simulink model "NE_Red_Rooster_Delta_B_28may"  (R2019b)
settings: Solver=FixedStepAuto  StartTime=0.0  StopTime=inf  FixedStep=0.0005  RelTol=1e-3
PreLoadFcn:
  | waijung.modelPreload; % Required for working with Waijung Blockset. Do not remove.
undefined symbols (not defined in the file): ARM, DiscIntNeverNeededParam, HSEOSC, Link, LQFP100, MDK, ST, STM32F407VG
libraries: simulink x30, stm32f4_i2c_lib x22, stm32f4_io_lib x6, stm32f4_reset_lib x1, stm32f4_device_config_lib x1
(part 4 of 5)

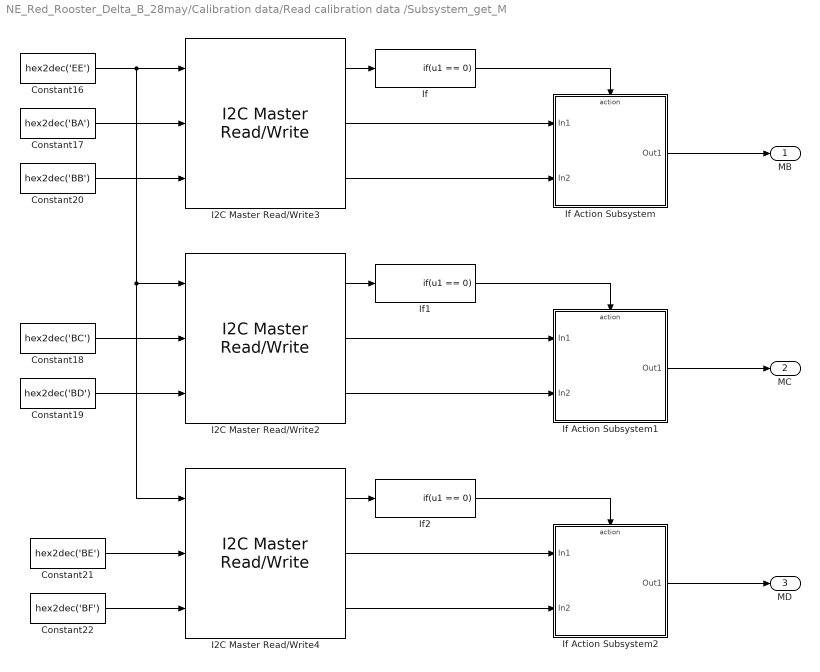
== system NE_Red_Rooster_Delta_B_28may/Calibration data/Read calibration data /Subsystem_get_M ==
  Constant16 : Constant  Value=hex2dec('EE')  OutDataTypeStr=uint8
  Constant17 : Constant  Value=hex2dec('BA')  OutDataTypeStr=uint8
  Constant18 : Constant  Value=hex2dec('BC')  OutDataTypeStr=uint8
  Constant19 : Constant  Value=hex2dec('BD')  OutDataTypeStr=uint8
  Constant20 : Constant  Value=hex2dec('BB')  OutDataTypeStr=uint8
  Constant21 : Constant  Value=hex2dec('BE')  OutDataTypeStr=uint8
  Constant22 : Constant  Value=hex2dec('BF')  OutDataTypeStr=uint8
  I2C Master Read/Write2 : stm32f4_i2c_lib/I2C Master Read//Write  configuration=Transaction  module=1  lastmodule=3  transfer=Blocking  dutycycle=TLow/THigh = 2  clkspeed=400  timeout=25  writecount=2  readcount=2  sdapin=C9  sclpin=A8  waitwritetime=0  forcestop=off  inputtypearray=[3 3 3 3]  outputtypearray=[3 3 3 3]  confstr="[\"C\",\"9\",\"A\",\"8\",\"1\",\"1\",\"6\",\"0\",\"I2C_DutyCycle_2\",\"0\",\"off\"]"  sampletime=-1  sampletimestr=Inf  blockid=CalibrationdataReadcalibrationdataSubsystem_get_MI2CMasterReadWrite2
  I2C Master Read/Write3 : stm32f4_i2c_lib/I2C Master Read//Write  configuration=Transaction  module=1  lastmodule=3  transfer=Blocking  dutycycle=TLow/THigh = 2  clkspeed=400  timeout=25  writecount=2  readcount=2  sdapin=C9  sclpin=A8  waitwritetime=0  forcestop=off  inputtypearray=[3 3 3 3]  outputtypearray=[3 3 3 3]  confstr="[\"C\",\"9\",\"A\",\"8\",\"1\",\"1\",\"6\",\"0\",\"I2C_DutyCycle_2\",\"0\",\"off\"]"  sampletime=-1  sampletimestr=Inf  blockid=CalibrationdataReadcalibrationdataSubsystem_get_MI2CMasterReadWrite3
  I2C Master Read/Write4 : stm32f4_i2c_lib/I2C Master Read//Write  configuration=Transaction  module=1  lastmodule=3  transfer=Blocking  dutycycle=TLow/THigh = 2  clkspeed=400  timeout=25  writecount=2  readcount=2  sdapin=C9  sclpin=A8  waitwritetime=0  forcestop=off  inputtypearray=[3 3 3 3]  outputtypearray=[3 3 3 3]  confstr="[\"C\",\"9\",\"A\",\"8\",\"1\",\"1\",\"6\",\"0\",\"I2C_DutyCycle_2\",\"0\",\"off\"]"  sampletime=-1  sampletimestr=Inf  blockid=CalibrationdataReadcalibrationdataSubsystem_get_MI2CMasterReadWrite4
  If : If  IfExpression=u1 == 0  ShowElse=off
  If Action Subsystem : Subsystem  TreatAsAtomicUnit=on
  If Action Subsystem1 : Subsystem  TreatAsAtomicUnit=on
  If Action Subsystem2 : Subsystem  TreatAsAtomicUnit=on
  If1 : If  IfExpression=u1 == 0  ShowElse=off
  If2 : If  IfExpression=u1 == 0  ShowElse=off
  MB : Outport
  MC : Outport  Port=2
  MD : Outport  Port=3
  wires:
  If Action Subsystem1/1(Out1) -> MC/1
  I2C Master Read/Write2/3 -> If Action Subsystem1/2(In2)
  I2C Master Read/Write3/1 -> If/1
  Constant16/1 -> I2C Master Read/Write4/1, I2C Master Read/Write2/1, I2C Master Read/Write3/1
  Constant22/1 -> I2C Master Read/Write4/3
  Constant21/1 -> I2C Master Read/Write4/2
  Constant20/1 -> I2C Master Read/Write3/3
  Constant18/1 -> I2C Master Read/Write2/2
  I2C Master Read/Write4/1 -> If2/1
  If1/1 -> If Action Subsystem1/Action
  If/1 -> If Action Subsystem/Action
  Constant19/1 -> I2C Master Read/Write2/3
  I2C Master Read/Write3/2 -> If Action Subsystem/1(In1)
  Constant17/1 -> I2C Master Read/Write3/2
  I2C Master Read/Write4/3 -> If Action Subsystem2/2(In2)
  I2C Master Read/Write3/3 -> If Action Subsystem/2(In2)
  If Action Subsystem/1(Out1) -> MB/1
  I2C Master Read/Write2/2 -> If Action Subsystem1/1(In1)
  I2C Master Read/Write4/2 -> If Action Subsystem2/1(In1)
  If Action Subsystem2/1(Out1) -> MD/1
  If2/1 -> If Action Subsystem2/Action
  I2C Master Read/Write2/1 -> If1/1

== system NE_Red_Rooster_Delta_B_28may/Init_L3GD4200 /Init L3G4200D/Subsystem ==
  Enable : EnablePort
  Logical Operator : Logic  Operator=NOT  AllPortsSameDT=off  OutDataTypeStr=boolean
  Memory : Memory  InheritSampleTime=on
  Out1 : Outport
  wires:
  Logical Operator/1 -> Out1/1, Memory/1
  Memory/1 -> Logical Operator/1

== system NE_Red_Rooster_Delta_B_28may/Init_L3GD4200 /Init L3G4200D/Subsystem1 ==
  Enable : EnablePort
  Logical Operator : Logic  Operator=NOT  AllPortsSameDT=off  OutDataTypeStr=boolean
  Memory : Memory  InheritSampleTime=on
  Out1 : Outport
  wires:
  Memory/1 -> Logical Operator/1
  Logical Operator/1 -> Memory/1, Out1/1

== system NE_Red_Rooster_Delta_B_28may/Orientation/Accelerometr/Manipulate Data ==
  LowAddress : Inport
  HighAddress : Inport  Port=2
  Add : Sum
  Data Type Conversion : DataTypeConversion  OutDataTypeStr=int16
  Data Type Conversion1 : DataTypeConversion  OutDataTypeStr=int16
  Shift Arithmetic1 : ArithShift  BitShiftNumber=8  BitShiftDirection=Left
  RawAccData : Outport
  wires:
  LowAddress/1 -> Data Type Conversion/1
  HighAddress/1 -> Data Type Conversion1/1
  Data Type Conversion/1 -> Add/1
  Data Type Conversion1/1 -> Shift Arithmetic1/1
  Shift Arithmetic1/1 -> Add/2
  Add/1 -> RawAccData/1

== system NE_Red_Rooster_Delta_B_28may/Orientation/Accelerometr/Manipulate Data1 ==
  LowAddress : Inport
  HighAddress : Inport  Port=2
  Add : Sum
  Data Type Conversion : DataTypeConversion  OutDataTypeStr=int16
  Data Type Conversion1 : DataTypeConversion  OutDataTypeStr=int16
  Shift Arithmetic1 : ArithShift  BitShiftNumber=8  BitShiftDirection=Left
  RawAccData : Outport
  wires:
  Add/1 -> RawAccData/1
  Shift Arithmetic1/1 -> Add/2
  Data Type Conversion1/1 -> Shift Arithmetic1/1
  Data Type Conversion/1 -> Add/1
  HighAddress/1 -> Data Type Conversion1/1
  LowAddress/1 -> Data Type Conversion/1

== system NE_Red_Rooster_Delta_B_28may/Orientation/Accelerometr/Manipulate Data2 ==
  LowAddress : Inport
  HighAddress : Inport  Port=2
  Add : Sum
  Data Type Conversion : DataTypeConversion  OutDataTypeStr=int16
  Data Type Conversion1 : DataTypeConversion  OutDataTypeStr=int16
  Shift Arithmetic1 : ArithShift  BitShiftNumber=8  BitShiftDirection=Left
  RawAccData : Outport
  wires:
  LowAddress/1 -> Data Type Conversion/1
  HighAddress/1 -> Data Type Conversion1/1
  Data Type Conversion/1 -> Add/1
  Data Type Conversion1/1 -> Shift Arithmetic1/1
  Shift Arithmetic1/1 -> Add/2
  Add/1 -> RawAccData/1

== system NE_Red_Rooster_Delta_B_28may/Orientation/Accelerometr/Subsystem ==
  Enable : EnablePort
  Logical Operator : Logic  Operator=NOT  AllPortsSameDT=off  OutDataTypeStr=boolean
  Memory : Memory  InheritSampleTime=on
  Out1 : Outport
  wires:
  Logical Operator/1 -> Out1/1, Memory/1
  Memory/1 -> Logical Operator/1

== system NE_Red_Rooster_Delta_B_28may/Orientation/Accelerometr/Subsystem1 ==
  Enable : EnablePort
  Logical Operator : Logic  Operator=NOT  AllPortsSameDT=off  OutDataTypeStr=boolean
  Memory : Memory  InheritSampleTime=on
  Out1 : Outport
  wires:
  Memory/1 -> Logical Operator/1
  Logical Operator/1 -> Memory/1, Out1/1

== system NE_Red_Rooster_Delta_B_28may/Orientation/Accelerometr/Subsystem2 ==
  Enable : EnablePort
  Logical Operator : Logic  Operator=NOT  AllPortsSameDT=off  OutDataTypeStr=boolean
  Memory : Memory  InheritSampleTime=on
  Out1 : Outport
  wires:
  Logical Operator/1 -> Out1/1, Memory/1
  Memory/1 -> Logical Operator/1

== system NE_Red_Rooster_Delta_B_28may/Orientation/Gyro/Data_transformation ==
  In1 : Inport
  In2 : Inport  Port=2
  In3 : Inport  Port=3
  Gain : Gain  Gain=5
  Gain1 : Gain  Gain=5
  Gain2 : Gain  Gain=5
  Subsystem : Subsystem
  Subsystem1 : Subsystem
  Subsystem2 : Subsystem
  Subsystem3 : Subsystem
  Out1 : Outport
  Out2 : Outport  Port=2
  Out3 : Outport  Port=3
  wires:
  Subsystem2/1(Out1) -> Out1/1
  Subsystem2/2(Out2) -> Out2/1
  Subsystem2/3(Out3) -> Out3/1
  In1/1 -> Subsystem/1(In1)
  In2/1 -> Subsystem1/1(In1)
  In3/1 -> Subsystem3/1(In1)
  Subsystem/1(Grad/sek) -> Gain/1
  Subsystem1/1(Grad/sek) -> Gain1/1
  Subsystem3/1(Grad/sek) -> Gain2/1
  Gain/1 -> Subsystem2/1(In1)
  Gain1/1 -> Subsystem2/2(In2)
  Gain2/1 -> Subsystem2/3(In3)

== system NE_Red_Rooster_Delta_B_28may/Orientation/Gyro/L3G4200D ==
  Read L3G4200D : Subsystem  TreatAsAtomicUnit=on
  SlvAddr1 : Constant  Value=hex2dec('D2')  OutDataTypeStr=uint8  SampleTime=-1
  Status : Outport
  X : Outport  Port=2
  Y : Outport  Port=3
  Z : Outport  Port=4
  wires:
  Read L3G4200D/4(OUT_Z) -> Z/1
  Read L3G4200D/3(OUT_Y) -> Y/1
  Read L3G4200D/2(OUT_X) -> X/1
  Read L3G4200D/1(Status) -> Status/1
  SlvAddr1/1 -> Read L3G4200D/1(SlvAddr)

== system NE_Red_Rooster_Delta_B_28may/Orientation/Gyro/Success ==
  In1 : Inport
  In2 : Inport  Port=2
  In3 : Inport  Port=3
  Enable : EnablePort  PropagateVarSize=During execution
  Data Type Conversion : DataTypeConversion  OutDataTypeStr=int16
  Demux : Demux  Outputs=3
  Gain : Gain  Gain=250/2^15  ParamDataTypeStr=single  OutDataTypeStr=single
  Mux : Mux  Inputs=3
  Gyr_X : Outport
  Gyr_Y : Outport  Port=2
  Gyr_Z : Outport  Port=3
  wires:
  Data Type Conversion/1 -> Gain/1
  In3/1 -> Mux/3
  In2/1 -> Mux/2
  In1/1 -> Mux/1
  Demux/3 -> Gyr_Z/1
  Demux/2 -> Gyr_Y/1
  Demux/1 -> Gyr_X/1
  Gain/1 -> Demux/1
  Mux/1 -> Data Type Conversion/1

== system NE_Red_Rooster_Delta_B_28may/Baro_Altimeter/Calculate true pressure and temp /Calculate true pressure1/Altitude ==
  In1 : Inport
  "Null_Pressure " : Inport  Port=2
  Constant : Constant  Value=44330  OutDataTypeStr=int32
  Constant1 : Constant  OutDataTypeStr=int32
  Constant2 : Constant  Value=0.19  OutDataTypeStr=double
  Constant3 : Constant  Value=102159
  Divide : Product  Inputs=*/  OutDataTypeStr=double
  Math Function : Math  Operator=pow  SaturateOnIntegerOverflow=on
  Product : Product  OutDataTypeStr=single
  Subtract : Sum  Inputs=+-  OutDataTypeStr=double
  Terminator : Terminator
  Out1 : Outport
  wires:
  Product/1 -> Out1/1
  Constant1/1 -> Subtract/1
  Constant/1 -> Product/2
  Constant2/1 -> Math Function/2
  Subtract/1 -> Product/1
  In1/1 -> Divide/1
  Divide/1 -> Math Function/1
  Math Function/1 -> Subtract/2
  "Null_Pressure "/1 -> Divide/2
  Constant3/1 -> Terminator/1

== system NE_Red_Rooster_Delta_B_28may/Baro_Altimeter/Calculate true pressure and temp /Calculate true pressure1/If Action Subsystem ==
  B7 : Inport
  B4 : Inport  Port=2
  Action Port : ActionPort  ActionPortLabel=if { }
  Constant : Constant  Value=2  OutDataTypeStr=uint32
  Divide : Product  Inputs=*/  OutDataTypeStr=uint32
  Product : Product  OutDataTypeStr=uint32
  p : Outport  OutDataTypeStr=uint32
  wires:
  B7/1 -> Product/1
  Constant/1 -> Product/2
  Product/1 -> Divide/1
  B4/1 -> Divide/2
  Divide/1 -> p/1

== system NE_Red_Rooster_Delta_B_28may/Baro_Altimeter/Calculate true pressure and temp /Calculate true pressure1/If Action Subsystem1 ==
  B7 : Inport
  B4 : Inport  Port=2
  Action Port : ActionPort  ActionPortLabel=else { }
  Constant : Constant  Value=2  OutDataTypeStr=uint32
  Divide : Product  Inputs=*/
  Product : Product  OutDataTypeStr=uint32
  p : Outport  OutDataTypeStr=uint32
  wires:
  Constant/1 -> Product/2
  B4/1 -> Divide/2
  B7/1 -> Divide/1
  Divide/1 -> Product/1
  Product/1 -> p/1

== system NE_Red_Rooster_Delta_B_28may/Baro_Altimeter/Calculate true pressure and temp /Calculate true pressure1/New X1 value ==
  note: Версия 1: Формула для вычисления X1 имела следующий вид:
      | X1=AC3*B6/2^13
      | Я сначало делил потом умножал...
      |
      | Версия 2: X1=(AC3*B6)/2^13. Теперь я умножаю,а потом делю
  B6 : Inport
  AC3 : Inport  Port=2
  Constant : Constant  Value=8192  OutDataTypeStr=int32
  Divide : Product  Inputs=*/
  Product : Product  OutDataTypeStr=int32
  X1_1 : Outport  OutDataTypeStr=int32
  wires:
  AC3/1 -> Product/1
  Constant/1 -> Divide/2
  Product/1 -> Divide/1
  B6/1 -> Product/2
  Divide/1 -> X1_1/1

== system NE_Red_Rooster_Delta_B_28may/Baro_Altimeter/Calculate true pressure and temp /Calculate true pressure1/New_X2 ==
  B6 : Inport
  B1 : Inport  Port=2
  Constant1 : Constant  Value=4096  OutDataTypeStr=int32
  Constant2 : Constant  Value=65536  OutDataTypeStr=int32
  Divide : Product  Inputs=*/  OutDataTypeStr=int32
  Divide1 : Product  Inputs=*/  OutDataTypeStr=int32
  Product : Product  OutDataTypeStr=int32
  Product1 : Product  OutDataTypeStr=int32
  X2_1 : Outport  OutDataTypeStr=int32
  wires:
  B1/1 -> Product1/2
  Constant1/1 -> Divide/2
  B6/1 -> Product/2, Product/1
  Product1/1 -> Divide1/1
  Constant2/1 -> Divide1/2
  Divide1/1 -> X2_1/1
  Product/1 -> Divide/1
  Divide/1 -> Product1/1

== system NE_Red_Rooster_Delta_B_28may/Baro_Altimeter/Calculate true pressure and temp /Calculate true pressure1/Sub ==
  B6 : Inport
  B2 : Inport  Port=2
  2e11 : Subsystem
  2e12 : Subsystem
  Divide : Product  Inputs=*/
  Divide1 : Product  Inputs=*/
  Math Function : Math  Operator=square  SaturateOnIntegerOverflow=on
  Product1 : Product
  X1 : Outport
  wires:
  Divide1/1 -> X1/1
  2e11/1(Out1) -> Divide1/2
  Product1/1 -> Divide1/1
  B6/1 -> Math Function/1
  2e12/1(Out1) -> Divide/2
  B2/1 -> Product1/2
  Math Function/1 -> Divide/1
  Divide/1 -> Product1/1

== system NE_Red_Rooster_Delta_B_28may/Baro_Altimeter/Calculate true pressure and temp /Calculate true pressure1/Subsystem ==
  B5 : Inport
  Constant : Constant  Value=4000  OutDataTypeStr=int32
  Subtract : Sum  Inputs=+-  OutDataTypeStr=int32
  B6 : Outport  OutDataTypeStr=int32
  wires:
  B5/1 -> Subtract/1
  Subtract/1 -> B6/1
  Constant/1 -> Subtract/2

== system NE_Red_Rooster_Delta_B_28may/Baro_Altimeter/Calculate true pressure and temp /Calculate true pressure1/Subsystem1 ==
  B6 : Inport
  AC2 : Inport  Port=2
  2e11 : Subsystem
  Divide : Product  Inputs=*/
  Product : Product
  X2 : Outport
  wires:
  B6/1 -> Divide/1
  Product/1 -> X2/1
  Divide/1 -> Product/2
  2e11/1(Out1) -> Divide/2
  AC2/1 -> Product/1

== system NE_Red_Rooster_Delta_B_28may/Baro_Altimeter/Calculate true pressure and temp /Calculate true pressure1/Subsystem2 ==
  note: В тестовом примере сдвиг равен нулю, а у нас 3, с этого момента начинает алгоритм плыть..
  X3 : Inport
  AC1 : Inport  Port=2
  Add1 : Sum  OutDataTypeStr=int32
  Add2 : Sum  AccumDataTypeStr=int32
  Constant : Constant  Value=4  OutDataTypeStr=int32
  Constant1 : Constant  Value=2  OutDataTypeStr=int32
  Constant2 : Constant  Value=4  OutDataTypeStr=int32
  Divide : Product  Inputs=*/  OutDataTypeStr=int32
  Product : Product  OutDataTypeStr=int32
  Shift Arithmetic7 : ArithShift  BitShiftNumber=3  BitShiftDirection=Left  DiagnosticForOORShift=Warning
  B3 : Outport  OutDataTypeStr=int32
  wires:
  X3/1 -> Add1/1
  Product/1 -> Add1/2
  Constant/1 -> Product/2
  Divide/1 -> B3/1
  Constant2/1 -> Divide/2
  Shift Arithmetic7/1 -> Add2/1
  Add1/1 -> Shift Arithmetic7/1
  Add2/1 -> Divide/1
  Constant1/1 -> Add2/2
  AC1/1 -> Product/1

== system NE_Red_Rooster_Delta_B_28may/Baro_Altimeter/Calculate true pressure and temp /Calculate true pressure1/Subsystem3 ==
  X1_1 : Inport
  X2_1 : Inport  Port=2
  Add1 : Sum
  Add2 : Sum  AccumDataTypeStr=int32
  Constant : Constant  Value=2  OutDataTypeStr=int32
  Constant1 : Constant  Value=4  OutDataTypeStr=int32
  Divide : Product  Inputs=*/  OutDataTypeStr=int32
  X3_1 : Outport  OutDataTypeStr=int32
  wires:
  Divide/1 -> X3_1/1
  X1_1/1 -> Add1/1
  Constant1/1 -> Divide/2
  Add2/1 -> Divide/1
  Constant/1 -> Add2/2
  X2_1/1 -> Add1/2
  Add1/1 -> Add2/1

== system NE_Red_Rooster_Delta_B_28may/Baro_Altimeter/Calculate true pressure and temp /Calculate true pressure1/Subsystem4 ==
  X3_1 : Inport
  AC4 : Inport  Port=2
  Add1 : Sum  OutDataTypeStr=uint32
  Constant : Constant  Value=32768  OutDataTypeStr=uint32
  Constant1 : Constant  Value=32768  OutDataTypeStr=uint32
  Divide : Product  Inputs=*/  OutDataTypeStr=uint32
  Product : Product  OutDataTypeStr=uint32
  B4 : Outport  OutDataTypeStr=uint32
  wires:
  AC4/1 -> Product/2
  X3_1/1 -> Add1/1
  Constant/1 -> Add1/2
  Constant1/1 -> Divide/2
  Add1/1 -> Product/1
  Product/1 -> Divide/1
  Divide/1 -> B4/1

== system NE_Red_Rooster_Delta_B_28may/Baro_Altimeter/Calculate true pressure and temp /Calculate true pressure1/Subsystem5 ==
  B3 : Inport
  UP : Inport  Port=2
  Constant : Constant  Value=50000  OutDataTypeStr=uint32
  Product : Product  OutDataTypeStr=uint32
  Shift Arithmetic7 : ArithShift  BitShiftNumber=2  BitShiftDirection=Right
  Subtract : Sum  Inputs=+-
  B7 : Outport  OutDataTypeStr=uint32
  wires:
  Constant/1 -> Shift Arithmetic7/1
  UP/1 -> Subtract/1
  Shift Arithmetic7/1 -> Product/2
  B3/1 -> Subtract/2
  Subtract/1 -> Product/1
  Product/1 -> B7/1

== system NE_Red_Rooster_Delta_B_28may/Baro_Altimeter/Calculate true pressure and temp /Calculate true pressure1/Subsystem6 ==
  p : Inport
  Constant : Constant  Value=256  OutDataTypeStr=uint32
  Constant1 : Constant  Value=256  OutDataTypeStr=uint32
  Divide : Product  Inputs=*/  OutDataTypeStr=uint32
  Divide1 : Product  Inputs=*/  OutDataTypeStr=uint32
  Product : Product  OutDataTypeStr=uint32
  X1 : Outport  OutDataTypeStr=uint32
  wires:
  Constant1/1 -> Divide1/2
  p/1 -> Divide1/1, Divide/1
  Constant/1 -> Divide/2
  Divide/1 -> Product/1
  Product/1 -> X1/1
  Divide1/1 -> Product/2

== system NE_Red_Rooster_Delta_B_28may/Baro_Altimeter/Calculate true pressure and temp /Calculate true pressure1/Subsystem7 ==
  X1 : Inport
  Constant : Constant  Value=3038  OutDataTypeStr=uint32
  Constant1 : Constant  Value=65536  OutDataTypeStr=uint32
  Divide : Product  Inputs=*/  OutDataTypeStr=uint32
  Product : Product
  X1_1 : Outport  OutDataTypeStr=uint32
  wires:
  X1/1 -> Product/1
  Product/1 -> Divide/1
  Constant1/1 -> Divide/2
  Divide/1 -> X1_1/1
  Constant/1 -> Product/2

== system NE_Red_Rooster_Delta_B_28may/Baro_Altimeter/Calculate true pressure and temp /Calculate true pressure1/Subsystem8 ==
  p : Inport
  Constant : Constant  Value=-7357  OutDataTypeStr=int32
  Constant1 : Constant  Value=65536  OutDataTypeStr=int32
  Divide : Product  Inputs=*/  OutDataTypeStr=int32
  Product : Product  OutDataTypeStr=int32
  X2 : Outport  OutDataTypeStr=int32
  wires:
  Product/1 -> Divide/1
  Constant1/1 -> Divide/2
  p/1 -> Product/1
  Divide/1 -> X2/1
  Constant/1 -> Product/2

== system NE_Red_Rooster_Delta_B_28may/Baro_Altimeter/Calculate true pressure and temp /Calculate true pressure1/Subsystem9 ==
  p : Inport
  X1_1 : Inport  Port=2
  X2 : Inport  Port=3
  Add1 : Sum  Inputs=+++  OutDataTypeStr=int32
  Add2 : Sum  OutDataTypeStr=int32
  Constant : Constant  Value=3791  OutDataTypeStr=uint32
  Constant1 : Constant  Value=16  OutDataTypeStr=uint32
  Divide : Product  Inputs=*/  OutDataTypeStr=int32
  p_1 : Outport  OutDataTypeStr=int32
  wires:
  X1_1/1 -> Add1/1
  X2/1 -> Add1/2
  Add1/1 -> Divide/1
  Constant/1 -> Add1/3
  Constant1/1 -> Divide/2
  Divide/1 -> Add2/2
  p/1 -> Add2/1
  Add2/1 -> p_1/1

== system NE_Red_Rooster_Delta_B_28may/Baro_Altimeter/Calculate true pressure and temp /Calculate true temperature1/Subsystem ==
  UT : Inport
  AC6 : Inport  Port=2
  AC5 : Inport  Port=3
  Add : Sum  Inputs=+-  OutDataTypeStr=int32
  Constant : Constant  Value=32768  OutDataTypeStr=int32
  Divide : Product  Inputs=*/  OutDataTypeStr=int32
  Product : Product
  X1 : Outport
  wires:
  AC6/1 -> Add/2
  UT/1 -> Add/1
  Add/1 -> Product/1
  Constant/1 -> Divide/2
  AC5/1 -> Product/2
  Product/1 -> Divide/1
  Divide/1 -> X1/1

== system NE_Red_Rooster_Delta_B_28may/Baro_Altimeter/Calculate true pressure and temp /Calculate true temperature1/Subsystem1 ==
  X1 : Inport
  MC : Inport  Port=2
  MD : Inport  Port=3
  Add : Sum
  Constant2 : Constant  Value=2048  OutDataTypeStr=int32
  Divide : Product  Inputs=*/  OutDataTypeStr=int32
  Product : Product  OutDataTypeStr=int32
  X2 : Outport
  wires:
  Divide/1 -> X2/1
  X1/1 -> Add/1
  Add/1 -> Divide/2
  MD/1 -> Add/2
  Product/1 -> Divide/1
  MC/1 -> Product/1
  Constant2/1 -> Product/2

== system NE_Red_Rooster_Delta_B_28may/Baro_Altimeter/Calculate true pressure and temp /Calculate true temperature1/Subsystem2 ==
  B5 : Inport
  Add1 : Sum  OutDataTypeStr=int32
  Constant : Constant  Value=8  OutDataTypeStr=uint32
  Constant1 : Constant  Value=16
  Divide : Product  Inputs=*/  OutDataTypeStr=int32
  T : Outport  OutDataTypeStr=int32
  wires:
  B5/1 -> Add1/1
  Add1/1 -> Divide/1
  Constant/1 -> Add1/2
  Constant1/1 -> Divide/2
  Divide/1 -> T/1

== system NE_Red_Rooster_Delta_B_28may/Baro_Altimeter/Read Pressure and Temp/If Action Subsystem/If Action Subsystem ==
  In1 : Inport
  Action Port : ActionPort  ActionPortLabel=if { }
  Data Type Conversion15 : DataTypeConversion  OutDataTypeStr=uint32
  Out1 : Outport
  wires:
  Data Type Conversion15/1 -> Out1/1
  In1/1 -> Data Type Conversion15/1

== system NE_Red_Rooster_Delta_B_28may/Baro_Altimeter/Read Pressure and Temp/If Action Subsystem/If Action Subsystem1 ==
  In1 : Inport
  Action Port : ActionPort  ActionPortLabel=if { }
  Constant : Constant  Value=16777216  OutDataTypeStr=uint32  SampleTime=-1
  Subtract : Sum  Inputs=+-  OutDataTypeStr=int32
  Out1 : Outport
  wires:
  In1/1 -> Subtract/1
  Subtract/1 -> Out1/1
  Constant/1 -> Subtract/2

== system NE_Red_Rooster_Delta_B_28may/Baro_Altimeter/Read Pressure and Temp/If Action Subsystem/If Action Subsystem2 ==
  In1 : Inport
  Action Port : ActionPort  ActionPortLabel=else { }
  Out1 : Outport
  wires:
  In1/1 -> Out1/1

== system NE_Red_Rooster_Delta_B_28may/Baro_Altimeter/Read Pressure and Temp/If Action Subsystem/If Action Subsystem3 ==
  In1 : Inport
  Action Port : ActionPort  ActionPortLabel=if { }
  Data Type Conversion15 : DataTypeConversion  OutDataTypeStr=uint32
  Out1 : Outport
  wires:
  Data Type Conversion15/1 -> Out1/1
  In1/1 -> Data Type Conversion15/1

== system NE_Red_Rooster_Delta_B_28may/Baro_Altimeter/Read Pressure and Temp/If Action Subsystem2/If Action Subsystem ==
  In1 : Inport
  Action Port : ActionPort  ActionPortLabel=if { }
  Data Type Conversion4 : DataTypeConversion  OutDataTypeStr=uint32
  Out1 : Outport
  wires:
  In1/1 -> Data Type Conversion4/1
  Data Type Conversion4/1 -> Out1/1

== system NE_Red_Rooster_Delta_B_28may/Baro_Altimeter/Read Pressure and Temp/If Action Subsystem2/If Action Subsystem1 ==
  In2 : Inport
  Action Port : ActionPort  ActionPortLabel=if { }
  Data Type Conversion1 : DataTypeConversion  OutDataTypeStr=uint32
  Out1 : Outport
  wires:
  In2/1 -> Data Type Conversion1/1
  Data Type Conversion1/1 -> Out1/1

== system NE_Red_Rooster_Delta_B_28may/Baro_Altimeter/Read Pressure and Temp/If Action Subsystem2/If Action Subsystem2 ==
  In2 : Inport
  Action Port : ActionPort  ActionPortLabel=if { }
  Data Type Conversion1 : DataTypeConversion  OutDataTypeStr=uint32
  Out1 : Outport
  wires:
  In2/1 -> Data Type Conversion1/1
  Data Type Conversion1/1 -> Out1/1

== system NE_Red_Rooster_Delta_B_28may/Calibration data/Read calibration data /Subsystem_get_AC/If Action Subsystem ==
  In1 : Inport
  In2 : Inport  Port=2
  Action Port : ActionPort  ActionPortLabel=if { }
  Add9 : Sum  AccumDataTypeStr=uint32  OutDataTypeStr=int32
  Compare To Constant : simulink/Logic and Bit Operations/Compare To Constant  relop=>=  const=128  OutDataTypeStr=boolean
  Data Type Conversion15 : DataTypeConversion  OutDataTypeStr=uint32
  Data Type Conversion16 : DataTypeConversion  OutDataTypeStr=uint32
  If : If  IfExpression=u1 >= 128
  If Action Subsystem : Subsystem  TreatAsAtomicUnit=on
  If Action Subsystem1 : Subsystem  TreatAsAtomicUnit=on
  Shift Arithmetic9 : ArithShift  BitShiftNumber=8  BitShiftDirection=Left
  Switch : Switch  Criteria=u2 > Threshold
  Out1 : Outport
  wires:
  Compare To Constant/1 -> Switch/2
  Switch/1 -> Out1/1
  If Action Subsystem1/1(Out1) -> Switch/3
  If Action Subsystem/1(Out1) -> Switch/1
  If/2 -> If Action Subsystem1/Action
  Add9/1 -> If Action Subsystem/1(In1), If Action Subsystem1/1(In1)
  If/1 -> If Action Subsystem/Action
  In2/1 -> Data Type Conversion16/1
  In1/1 -> Data Type Conversion15/1
  Data Type Conversion15/1 -> Shift Arithmetic9/1, If/1, Compare To Constant/1
  Data Type Conversion16/1 -> Add9/2
  Shift Arithmetic9/1 -> Add9/1

== system NE_Red_Rooster_Delta_B_28may/Calibration data/Read calibration data /Subsystem_get_AC/If Action Subsystem1 ==
  In1 : Inport
  In2 : Inport  Port=2
  Action Port : ActionPort  ActionPortLabel=if { }
  Add9 : Sum  AccumDataTypeStr=uint32  OutDataTypeStr=int32
  Compare To Constant : simulink/Logic and Bit Operations/Compare To Constant  relop=>=  const=128  OutDataTypeStr=boolean
  Data Type Conversion15 : DataTypeConversion  OutDataTypeStr=uint32
  Data Type Conversion16 : DataTypeConversion  OutDataTypeStr=uint32
  If : If  IfExpression=u1 >= 128
  If Action Subsystem : Subsystem  TreatAsAtomicUnit=on
  If Action Subsystem1 : Subsystem  TreatAsAtomicUnit=on
  Shift Arithmetic9 : ArithShift  BitShiftNumber=8  BitShiftDirection=Left
  Switch : Switch  Criteria=u2 > Threshold
  Out1 : Outport
  wires:
  Compare To Constant/1 -> Switch/2
  Switch/1 -> Out1/1
  If Action Subsystem1/1(Out1) -> Switch/3
  If Action Subsystem/1(Out1) -> Switch/1
  If/2 -> If Action Subsystem1/Action
  Add9/1 -> If Action Subsystem/1(In1), If Action Subsystem1/1(In1)
  If/1 -> If Action Subsystem/Action
  In2/1 -> Data Type Conversion16/1
  In1/1 -> Data Type Conversion15/1
  Data Type Conversion15/1 -> Shift Arithmetic9/1, If/1, Compare To Constant/1
  Data Type Conversion16/1 -> Add9/2
  Shift Arithmetic9/1 -> Add9/1

== system NE_Red_Rooster_Delta_B_28may/Calibration data/Read calibration data /Subsystem_get_AC/If Action Subsystem2 ==
  In1 : Inport
  In2 : Inport  Port=2
  Action Port : ActionPort  ActionPortLabel=if { }
  Add9 : Sum  AccumDataTypeStr=uint32  OutDataTypeStr=int32
  Compare To Constant : simulink/Logic and Bit Operations/Compare To Constant  relop=>=  const=128  OutDataTypeStr=boolean
  Data Type Conversion15 : DataTypeConversion  OutDataTypeStr=uint32
  Data Type Conversion16 : DataTypeConversion  OutDataTypeStr=uint32
  If : If  IfExpression=u1 >= 128
  If Action Subsystem : Subsystem  TreatAsAtomicUnit=on
  If Action Subsystem1 : Subsystem  TreatAsAtomicUnit=on
  Shift Arithmetic9 : ArithShift  BitShiftNumber=8  BitShiftDirection=Left
  Switch : Switch  Criteria=u2 > Threshold
  Out1 : Outport
  wires:
  Compare To Constant/1 -> Switch/2
  Switch/1 -> Out1/1
  If Action Subsystem1/1(Out1) -> Switch/3
  If Action Subsystem/1(Out1) -> Switch/1
  If/2 -> If Action Subsystem1/Action
  Add9/1 -> If Action Subsystem/1(In1), If Action Subsystem1/1(In1)
  If/1 -> If Action Subsystem/Action
  In2/1 -> Data Type Conversion16/1
  In1/1 -> Data Type Conversion15/1
  Data Type Conversion15/1 -> Shift Arithmetic9/1, If/1, Compare To Constant/1
  Data Type Conversion16/1 -> Add9/2
  Shift Arithmetic9/1 -> Add9/1

== system NE_Red_Rooster_Delta_B_28may/Calibration data/Read calibration data /Subsystem_get_AC/If Action Subsystem3 ==
  In1 : Inport
  In2 : Inport  Port=2
  Action Port : ActionPort  ActionPortLabel=if { }
  Add9 : Sum  AccumDataTypeStr=uint32  OutDataTypeStr=uint32
  Data Type Conversion15 : DataTypeConversion  OutDataTypeStr=uint32
  Data Type Conversion16 : DataTypeConversion  OutDataTypeStr=uint32
  Shift Arithmetic9 : ArithShift  BitShiftNumber=8  BitShiftDirection=Left
  Out1 : Outport
  wires:
  In2/1 -> Data Type Conversion16/1
  In1/1 -> Data Type Conversion15/1
  Data Type Conversion15/1 -> Shift Arithmetic9/1
  Data Type Conversion16/1 -> Add9/2
  Shift Arithmetic9/1 -> Add9/1
  Add9/1 -> Out1/1

== system NE_Red_Rooster_Delta_B_28may/Calibration data/Read calibration data /Subsystem_get_AC/If Action Subsystem4 ==
  In1 : Inport
  In2 : Inport  Port=2
  Action Port : ActionPort  ActionPortLabel=if { }
  Add9 : Sum  AccumDataTypeStr=uint32  OutDataTypeStr=uint32
  Data Type Conversion15 : DataTypeConversion  OutDataTypeStr=uint32
  Data Type Conversion16 : DataTypeConversion  OutDataTypeStr=uint32
  Shift Arithmetic9 : ArithShift  BitShiftNumber=8  BitShiftDirection=Left
  Out1 : Outport
  wires:
  In2/1 -> Data Type Conversion16/1
  In1/1 -> Data Type Conversion15/1
  Data Type Conversion15/1 -> Shift Arithmetic9/1
  Data Type Conversion16/1 -> Add9/2
  Shift Arithmetic9/1 -> Add9/1
  Add9/1 -> Out1/1

== system NE_Red_Rooster_Delta_B_28may/Calibration data/Read calibration data /Subsystem_get_AC/If Action Subsystem5 ==
  In1 : Inport
  In2 : Inport  Port=2
  Action Port : ActionPort  ActionPortLabel=if { }
  Add9 : Sum  AccumDataTypeStr=uint32  OutDataTypeStr=uint32
  Data Type Conversion15 : DataTypeConversion  OutDataTypeStr=uint32
  Data Type Conversion16 : DataTypeConversion  OutDataTypeStr=uint32
  Shift Arithmetic9 : ArithShift  BitShiftNumber=8  BitShiftDirection=Left
  Out1 : Outport
  wires:
  In2/1 -> Data Type Conversion16/1
  In1/1 -> Data Type Conversion15/1
  Data Type Conversion15/1 -> Shift Arithmetic9/1
  Data Type Conversion16/1 -> Add9/2
  Shift Arithmetic9/1 -> Add9/1
  Add9/1 -> Out1/1

== system NE_Red_Rooster_Delta_B_28may/Calibration data/Read calibration data /Subsystem_get_B/If Action Subsystem ==
  In1 : Inport
  In2 : Inport  Port=2
  Action Port : ActionPort  ActionPortLabel=if { }
  Add9 : Sum  AccumDataTypeStr=uint32  OutDataTypeStr=int32
  Compare To Constant : simulink/Logic and Bit Operations/Compare To Constant  relop=>=  const=128  OutDataTypeStr=boolean
  Data Type Conversion15 : DataTypeConversion  OutDataTypeStr=uint32
  Data Type Conversion16 : DataTypeConversion  OutDataTypeStr=uint32
  If : If  IfExpression=u1 >= 128
  If Action Subsystem : Subsystem  TreatAsAtomicUnit=on
  If Action Subsystem1 : Subsystem  TreatAsAtomicUnit=on
  Shift Arithmetic9 : ArithShift  BitShiftNumber=8  BitShiftDirection=Left
  Switch : Switch  Criteria=u2 > Threshold
  Out1 : Outport
  wires:
  Compare To Constant/1 -> Switch/2
  Switch/1 -> Out1/1
  If Action Subsystem1/1(Out1) -> Switch/3
  If Action Subsystem/1(Out1) -> Switch/1
  If/2 -> If Action Subsystem1/Action
  Add9/1 -> If Action Subsystem/1(In1), If Action Subsystem1/1(In1)
  If/1 -> If Action Subsystem/Action
  In2/1 -> Data Type Conversion16/1
  In1/1 -> Data Type Conversion15/1
  Data Type Conversion15/1 -> Shift Arithmetic9/1, If/1, Compare To Constant/1
  Data Type Conversion16/1 -> Add9/2
  Shift Arithmetic9/1 -> Add9/1

== system NE_Red_Rooster_Delta_B_28may/Calibration data/Read calibration data /Subsystem_get_B/If Action Subsystem1 ==
  In1 : Inport
  In2 : Inport  Port=2
  Action Port : ActionPort  ActionPortLabel=if { }
  Add9 : Sum  AccumDataTypeStr=uint32  OutDataTypeStr=int32
  Compare To Constant : simulink/Logic and Bit Operations/Compare To Constant  relop=>=  const=128  OutDataTypeStr=boolean
  Data Type Conversion15 : DataTypeConversion  OutDataTypeStr=uint32
  Data Type Conversion16 : DataTypeConversion  OutDataTypeStr=uint32
  If : If  IfExpression=u1 >= 128
  If Action Subsystem : Subsystem  TreatAsAtomicUnit=on
  If Action Subsystem1 : Subsystem  TreatAsAtomicUnit=on
  Shift Arithmetic9 : ArithShift  BitShiftNumber=8  BitShiftDirection=Left
  Switch : Switch  Criteria=u2 > Threshold
  Out1 : Outport
  wires:
  Compare To Constant/1 -> Switch/2
  Switch/1 -> Out1/1
  If Action Subsystem1/1(Out1) -> Switch/3
  If Action Subsystem/1(Out1) -> Switch/1
  If/2 -> If Action Subsystem1/Action
  Add9/1 -> If Action Subsystem/1(In1), If Action Subsystem1/1(In1)
  If/1 -> If Action Subsystem/Action
  In2/1 -> Data Type Conversion16/1
  In1/1 -> Data Type Conversion15/1
  Data Type Conversion15/1 -> Shift Arithmetic9/1, If/1, Compare To Constant/1
  Data Type Conversion16/1 -> Add9/2
  Shift Arithmetic9/1 -> Add9/1

== system NE_Red_Rooster_Delta_B_28may/Calibration data/Read calibration data /Subsystem_get_M/If Action Subsystem ==
  In1 : Inport
  In2 : Inport  Port=2
  Action Port : ActionPort  ActionPortLabel=if { }
  Add9 : Sum  AccumDataTypeStr=uint32  OutDataTypeStr=int32
  Compare To Constant : simulink/Logic and Bit Operations/Compare To Constant  relop=>=  const=128  OutDataTypeStr=boolean
  Data Type Conversion15 : DataTypeConversion  OutDataTypeStr=uint32
  Data Type Conversion16 : DataTypeConversion  OutDataTypeStr=uint32
  If : If  IfExpression=u1 >= 128
  If Action Subsystem : Subsystem  TreatAsAtomicUnit=on
  If Action Subsystem1 : Subsystem  TreatAsAtomicUnit=on
  Shift Arithmetic9 : ArithShift  BitShiftNumber=8  BitShiftDirection=Left
  Switch : Switch  Criteria=u2 > Threshold
  Out1 : Outport
  wires:
  Shift Arithmetic9/1 -> Add9/1
  Data Type Conversion16/1 -> Add9/2
  Data Type Conversion15/1 -> Compare To Constant/1, If/1, Shift Arithmetic9/1
  In1/1 -> Data Type Conversion15/1
  In2/1 -> Data Type Conversion16/1
  If/1 -> If Action Subsystem/Action
  Add9/1 -> If Action Subsystem1/1(In1), If Action Subsystem/1(In1)
  If/2 -> If Action Subsystem1/Action
  If Action Subsystem/1(Out1) -> Switch/1
  If Action Subsystem1/1(Out1) -> Switch/3
  Switch/1 -> Out1/1
  Compare To Constant/1 -> Switch/2

== system NE_Red_Rooster_Delta_B_28may/Calibration data/Read calibration data /Subsystem_get_M/If Action Subsystem1 ==
  In1 : Inport
  In2 : Inport  Port=2
  Action Port : ActionPort  ActionPortLabel=if { }
  Add9 : Sum  AccumDataTypeStr=uint32  OutDataTypeStr=int32
  Compare To Constant : simulink/Logic and Bit Operations/Compare To Constant  relop=>=  const=128  OutDataTypeStr=boolean
  Data Type Conversion15 : DataTypeConversion  OutDataTypeStr=uint32
  Data Type Conversion16 : DataTypeConversion  OutDataTypeStr=uint32
  If : If  IfExpression=u1 >= 128
  If Action Subsystem : Subsystem  TreatAsAtomicUnit=on
  If Action Subsystem1 : Subsystem  TreatAsAtomicUnit=on
  Shift Arithmetic9 : ArithShift  BitShiftNumber=8  BitShiftDirection=Left
  Switch : Switch  Criteria=u2 > Threshold
  Out1 : Outport
  wires:
  Shift Arithmetic9/1 -> Add9/1
  Data Type Conversion16/1 -> Add9/2
  Data Type Conversion15/1 -> Compare To Constant/1, If/1, Shift Arithmetic9/1
  In1/1 -> Data Type Conversion15/1
  In2/1 -> Data Type Conversion16/1
  If/1 -> If Action Subsystem/Action
  Add9/1 -> If Action Subsystem1/1(In1), If Action Subsystem/1(In1)
  If/2 -> If Action Subsystem1/Action
  If Action Subsystem/1(Out1) -> Switch/1
  If Action Subsystem1/1(Out1) -> Switch/3
  Switch/1 -> Out1/1
  Compare To Constant/1 -> Switch/2

== system NE_Red_Rooster_Delta_B_28may/Calibration data/Read calibration data /Subsystem_get_M/If Action Subsystem2 ==
  In1 : Inport
  In2 : Inport  Port=2
  Action Port : ActionPort  ActionPortLabel=if { }
  Add9 : Sum  AccumDataTypeStr=uint32  OutDataTypeStr=int32
  Compare To Constant : simulink/Logic and Bit Operations/Compare To Constant  relop=>=  const=128  OutDataTypeStr=boolean
  Data Type Conversion15 : DataTypeConversion  OutDataTypeStr=uint32
  Data Type Conversion16 : DataTypeConversion  OutDataTypeStr=uint32
  If : If  IfExpression=u1 >= 128
  If Action Subsystem : Subsystem  TreatAsAtomicUnit=on
  If Action Subsystem1 : Subsystem  TreatAsAtomicUnit=on
  Shift Arithmetic9 : ArithShift  BitShiftNumber=8  BitShiftDirection=Left
  Switch : Switch  Criteria=u2 > Threshold
  Out1 : Outport
  wires:
  Shift Arithmetic9/1 -> Add9/1
  Data Type Conversion16/1 -> Add9/2
  Data Type Conversion15/1 -> Compare To Constant/1, If/1, Shift Arithmetic9/1
  In1/1 -> Data Type Conversion15/1
  In2/1 -> Data Type Conversion16/1
  If/1 -> If Action Subsystem/Action
  Add9/1 -> If Action Subsystem1/1(In1), If Action Subsystem/1(In1)
  If/2 -> If Action Subsystem1/Action
  If Action Subsystem/1(Out1) -> Switch/1
  If Action Subsystem1/1(Out1) -> Switch/3
  Switch/1 -> Out1/1
  Compare To Constant/1 -> Switch/2

== system NE_Red_Rooster_Delta_B_28may/Orientation/Gyro/Data_transformation/Subsystem ==
  In1 : Inport
  Constant : Constant  Value=17.5
  Constant1 : Constant  Value=1000
  Divide : Product  Inputs=*/
  Product : Product
  Grad/sek : Outport
  wires:
  Constant1/1 -> Divide/2
  Product/1 -> Divide/1
  Constant/1 -> Product/2
  In1/1 -> Product/1
  Divide/1 -> Grad/sek/1

== system NE_Red_Rooster_Delta_B_28may/Orientation/Gyro/Data_transformation/Subsystem1 ==
  In1 : Inport
  Constant : Constant  Value=17.5
  Constant1 : Constant  Value=1000
  Divide : Product  Inputs=*/
  Product : Product
  Grad/sek : Outport
  wires:
  Divide/1 -> Grad/sek/1
  In1/1 -> Product/1
  Constant/1 -> Product/2
  Product/1 -> Divide/1
  Constant1/1 -> Divide/2

== system NE_Red_Rooster_Delta_B_28may/Orientation/Gyro/Data_transformation/Subsystem2 ==
  In1 : Inport
  In2 : Inport  Port=2
  In3 : Inport  Port=3
  Data Type Conversion : DataTypeConversion  OutDataTypeStr=single
  Data Type Conversion1 : DataTypeConversion  OutDataTypeStr=single
  Data Type Conversion2 : DataTypeConversion  OutDataTypeStr=single
  From_free_data_to_Angle : Subsystem
  Out1 : Outport
  Out2 : Outport  Port=2
  Out3 : Outport  Port=3
  wires:
  In1/1 -> From_free_data_to_Angle/3(W_Roll)
  From_free_data_to_Angle/1(Angle_Yaw) -> Data Type Conversion2/1
  From_free_data_to_Angle/2(Angle_Pitch) -> Data Type Conversion1/1
  From_free_data_to_Angle/3(Angle_Roll) -> Data Type Conversion/1
  In2/1 -> From_free_data_to_Angle/2(W_Pitch)
  In3/1 -> From_free_data_to_Angle/1(W_Yaw)
  Data Type Conversion/1 -> Out3/1
  Data Type Conversion1/1 -> Out2/1
  Data Type Conversion2/1 -> Out1/1

== system NE_Red_Rooster_Delta_B_28may/Orientation/Gyro/Data_transformation/Subsystem3 ==
  In1 : Inport
  Constant : Constant  Value=17.5
  Constant1 : Constant  Value=1000
  Divide : Product  Inputs=*/
  Product : Product
  Grad/sek : Outport
  wires:
  Constant1/1 -> Divide/2
  Product/1 -> Divide/1
  Constant/1 -> Product/2
  In1/1 -> Product/1
  Divide/1 -> Grad/sek/1
